simulink model "chap9_4"  (Simulink 3.00)
settings: Solver=ode45  StartTime=0.0  StopTime=3  RelTol=1e-3
settings Model: LastModifiedBy=Administrator

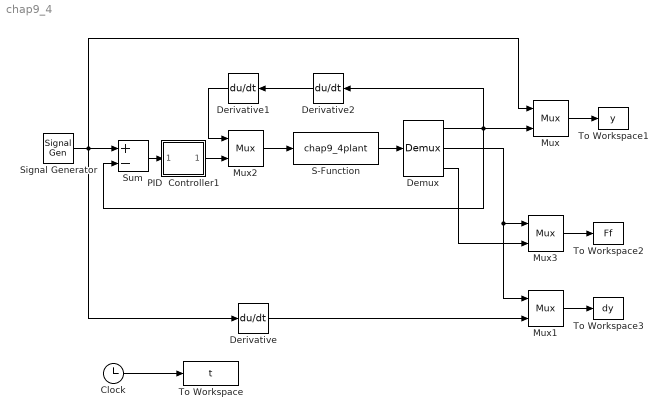
== system chap9_4 ==
  Clock : Clock
      settings: DisplayTime=off  Decimation=10
  Demux : Demux  Outputs=3
  Derivative : Derivative
  Derivative1 : Derivative  Orientation=left
  Derivative2 : Derivative  Orientation=left
  Mux{,1..3} (4 alike) : Mux  Inputs=2
      settings: DisplayOption=none
  PID  Controller1 : Subsystem  mask(PID Controller){@1=200, @2=0, @3=40}
      mask prompts: @1 "Proportional:"; @2 "Integral"; @3 "Derivative:"
      mask help:
      | Enter expressions for proportional, integral, and derivative terms.
      | P+I/s+Ds
      mask init:
      | P=@1; I=@2; D=@3;
      mask Help: This block implements a PID controller where parameters are entered for the Proportional, Integral and Derivative terms. Unmask this block to see how it works. The derivative term is implemented using a true derivative block.
      mask Display: disp('PID')
  S-Function : S-Function  FunctionName=chap9_4plant  PortCounts=[]  SFunctionModules=''
  Signal Generator : SignalGenerator  WaveForm=sine  Amplitude=0.1  Frequency=1  Units=Hertz
  Sum : Sum  Inputs=+-  SaturateOnIntegerOverflow=on
  To Workspace : ToWorkspace  VariableName=t  SampleTime=-1  SaveFormat=Matrix
  To Workspace1 : ToWorkspace  VariableName=y  SampleTime=-1  SaveFormat=Matrix
  To Workspace2 : ToWorkspace  VariableName=Ff  SampleTime=-1  SaveFormat=Matrix
  To Workspace3 : ToWorkspace  VariableName=dy  SampleTime=-1  SaveFormat=Matrix
  wires:
  Sum/1 -> PID  Controller1/1(In_1)
  S-Function/1 -> Demux/1
  Mux/1 -> To Workspace1/1
  Demux/1 -> Mux/2, Sum/2, Derivative2/1
  Mux2/1 -> S-Function/1
  PID  Controller1/1(Out_1) -> Mux2/2
  Derivative1/1 -> Mux2/1
  Derivative2/1 -> Derivative1/1
  Demux/3 -> Mux3/2
  Demux/2 -> Mux1/1, Mux3/1
  Mux3/1 -> To Workspace2/1
  Mux1/1 -> To Workspace3/1
  Derivative/1 -> Mux1/2
  Signal Generator/1 -> Sum/1, Mux/1, Derivative/1
  Clock/1 -> To Workspace/1

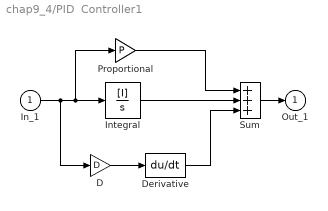
== system chap9_4/PID  Controller1 ==
  In_1 : Inport  Port=1  PortWidth=-1  SampleTime=-1  DataType=auto
      settings: SignalType=auto
  D : Gain  Gain=D  SaturateOnIntegerOverflow=on
  Derivative : Derivative
  Integral : TransferFcn  Numerator=[I]  Denominator=[1 0]
  Proportional : Gain  Gain=P  SaturateOnIntegerOverflow=on
  Sum : Sum  Inputs=+++  SaturateOnIntegerOverflow=on
  Out_1 : Outport  Port=1  InitialOutput=0
  wires:
  D/1 -> Derivative/1
  Sum/1 -> Out_1/1
  In_1/1 -> D/1, Proportional/1, Integral/1
  Derivative/1 -> Sum/3
  Integral/1 -> Sum/2
  Proportional/1 -> Sum/1
